simulink model "tt_sim"  (R2018b)
settings: Solver=FixedStepAuto  StartTime=0.0  StopTime=400  FixedStep=0.0001  RelTol=1e-5  EnableMultiTasking=on
StopFcn:
  | %e_unicycle_3d_trefoil_plot
libraries: simulink x2
settings Model: Creator=winston  LastModifiedBy=winston
settings SolverCC: AutoInsertRateTranBlk=on
settings DataIOCC: SaveOutput=off  SignalLogging=off  DSMLogging=off  SaveTime=off
settings OptimizationCC: LifeSpan=inf
settings DebuggingCC: AllowSymbolicDim=off  LibraryContextMissingDiagnostic=none  SFUnexpectedBacktrackingDiag=warning  SFNoUnconditionalDefaultTransitionDiag=warning  SFExecutionAtInitializationDiag=none  UnderSpecifiedDimensionMsg=warning
settings ModelReferenceCC: PropagateSignalLabelsOutOfModel=off
settings SFSimCC: SimUseLocalCustomCode=off
settings RTWCC: RTWUseLocalCustomCode=off
settings CodeAppCC: StateflowObjectComments=on
settings GRTTargetCC: TargetLangStandard=C89/C90 (ANSI)
settings ConfigComp: CovMetricSettings=dw  CovHtmlReporting=on  CovSaveCumulativeToWorkspaceVar=on  CovSaveSingleToWorkspaceVar=on  CovExternalEMLEnable=off

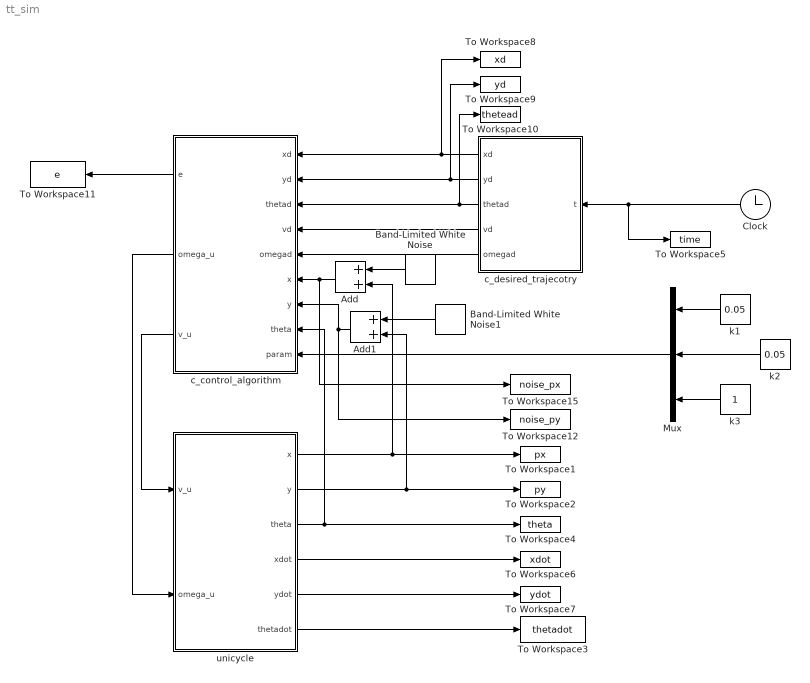
== system tt_sim ==
  Add : Sum
  Add1 : Sum
  Band-Limited White Noise : simulink/Sources/Band-Limited White Noise  Cov=10  Ts=0.1  seed=[23341]
  Band-Limited White Noise1 : simulink/Sources/Band-Limited White Noise  Cov=10  Ts=0.1  seed=[23]
  Clock : Clock
  Mux : Mux  Inputs=3
  To Workspace1 : ToWorkspace  VariableName=px  SampleTime=-1
  To Workspace10 : ToWorkspace  VariableName=thetead  SampleTime=-1
  To Workspace11 : ToWorkspace  VariableName=e  SaveFormat=Timeseries  SampleTime=-1
  To Workspace12 : ToWorkspace  VariableName=noise_py  SampleTime=-1
  To Workspace15 : ToWorkspace  VariableName=noise_px  SampleTime=-1
  To Workspace2 : ToWorkspace  VariableName=py  SampleTime=-1
  To Workspace3 : ToWorkspace  VariableName=thetadot  SampleTime=-1
  To Workspace4 : ToWorkspace  VariableName=theta  SampleTime=-1
  To Workspace5 : ToWorkspace  VariableName=time  SampleTime=-1
  To Workspace6 : ToWorkspace  VariableName=xdot  SampleTime=-1
  To Workspace7 : ToWorkspace  VariableName=ydot  SampleTime=-1
  To Workspace8 : ToWorkspace  VariableName=xd  SampleTime=-1
  To Workspace9 : ToWorkspace  VariableName=yd  SampleTime=-1
  c_control_algorithm : MATLAB Function  TreatAsAtomicUnit=on
  c_desired_trajecotry : MATLAB Function  TreatAsAtomicUnit=on
  k1 : Constant  Value=0.05
  k2 : Constant  Value=0.05
  k3 : Constant
  unicycle : Subsystem  mask{x0=300, y0=300, theta0=0}
      mask prompts: x0 "x(0)"; y0 "y(0)"; theta0 "theta(0)"
  wires:
  Mux/1 -> c_control_algorithm/9(param)
  c_control_algorithm/3(v_u) -> unicycle/1(v_u)
  c_control_algorithm/2(omega_u) -> unicycle/2(omega_u)
  k1/1 -> Mux/1
  k2/1 -> Mux/2
  k3/1 -> Mux/3
  Clock/1 -> To Workspace5/1, c_desired_trajecotry/1(t)
  unicycle/3(theta) -> c_control_algorithm/8(theta), To Workspace4/1
  unicycle/4(xdot) -> To Workspace6/1
  unicycle/5(ydot) -> To Workspace7/1
  unicycle/6(thetadot) -> To Workspace3/1
  c_desired_trajecotry/1(xd) -> c_control_algorithm/1(xd), To Workspace8/1
  c_desired_trajecotry/2(yd) -> c_control_algorithm/2(yd), To Workspace9/1
  c_desired_trajecotry/3(thetad) -> To Workspace10/1, c_control_algorithm/3(thetad)
  c_desired_trajecotry/4(vd) -> c_control_algorithm/4(vd)
  c_desired_trajecotry/5(omegad) -> c_control_algorithm/5(omegad)
  c_control_algorithm/1(e) -> To Workspace11/1
  unicycle/1(x) -> Add/2, To Workspace1/1
  Band-Limited White Noise/1 -> Add/1
  Add/1 -> To Workspace15/1, c_control_algorithm/6(x)
  unicycle/2(y) -> Add1/2, To Workspace2/1
  Band-Limited White Noise1/1 -> Add1/1
  Add1/1 -> c_control_algorithm/7(y), To Workspace12/1

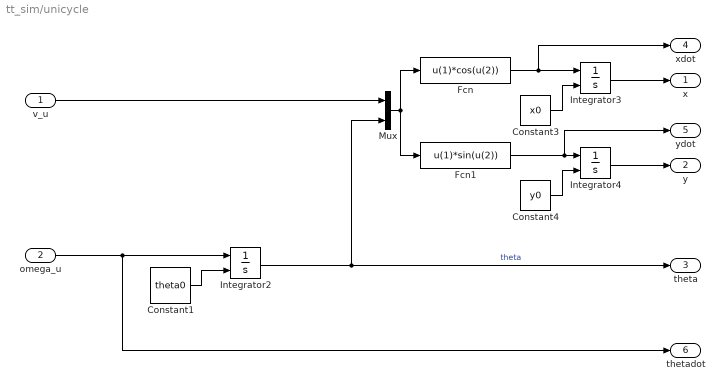
== system tt_sim/unicycle ==
  v_u : Inport
  omega_u : Inport  Port=2
  Constant1 : Constant  Value=theta0
  Constant3 : Constant  Value=x0
  Constant4 : Constant  Value=y0
  Fcn : Fcn  Expr=u(1)*cos(u(2))
  Fcn1 : Fcn  Expr=u(1)*sin(u(2))
  Integrator2 : Integrator  InitialConditionSource=external
  Integrator3 : Integrator  InitialConditionSource=external
  Integrator4 : Integrator  InitialConditionSource=external
  Mux : Mux  Inputs=2
  x : Outport
  y : Outport  Port=2
  theta : Outport  Port=3
  xdot : Outport  Port=4
  ydot : Outport  Port=5
  thetadot : Outport  Port=6
  wires:
  v_u/1 -> Mux/1
  Integrator2/1 -> theta/1, Mux/2  "theta"
  Mux/1 -> Fcn/1, Fcn1/1
  Fcn/1 -> xdot/1, Integrator3/1
  Fcn1/1 -> ydot/1, Integrator4/1
  Constant1/1 -> Integrator2/2
  Constant3/1 -> Integrator3/2
  Constant4/1 -> Integrator4/2
  omega_u/1 -> thetadot/1, Integrator2/1
  Integrator3/1 -> x/1
  Integrator4/1 -> y/1

== matlab function tt_sim/c_control_algorithm ==
  data: e output; omega_u output; xd input; yd input; thetad input; vd input; omegad input; v_u output; x input; y input; theta input; param input
function [e, omega_u, v_u] = fcn(xd, yd, thetad, vd, omegad, x, y, theta, param)
k1 = param(1); k2 = param(2); k3 = param(3);

M = [cos(theta), sin(theta), 0;
    -sin(theta), cos(theta), 0;
    0,           0         , 1];
e = M * [xd-x; yd-y; thetad-theta];

u1 = -k1*e(1);

tmp = sin(e(3))/e(3);
if(e(3) < 0.01)
    tmp = 1;
end
u2 = -k2*vd*e(2)*tmp - k3*e(3);

v_u = vd*cos(e(3)) - u1;
omega_u = omegad - u2;

== matlab function tt_sim/c_desired_trajecotry ==
  settings: updateMethod=DISCRETE
  data: t input; xd output; yd output; thetad output; vd output; omegad output
function [xd, yd, thetad, vd, omegad] = fcn(t)
persistent last_thetad
persistent unwrap_num
if isempty(last_thetad)
        last_thetad = 0;
end
if isempty(unwrap_num)
        unwrap_num = 0;
end

gain = 1/50; nx=3; ny=4; betax=0.1; betay=0.7;
xd = 250*cos(gain*nx*t+betax)+600;
yd = 250*cos(gain*ny*t+betay)+350;

dotxd = -15*sin((3*t)/50 + 1/10);
dotyd = -20*sin((2*t)/25 + 7/10);
thetad = atan2(dotyd, dotxd) + unwrap_num*2*pi;

% this part is to prevent discontinuity of atant2
if(thetad - last_thetad > pi)
    thetad = thetad-2*pi;
    unwrap_num = unwrap_num-1;
else
    if((thetad - last_thetad < -pi))
        thetad = thetad+2*pi;
        unwrap_num = unwrap_num+1;
    end
end
last_thetad = thetad;

vd = 5*(16*sin((2*t)/25 + 7/10)^2 + 9*sin((3*t)/50 + 1/10)^2)^(1/2);
omegad = (42*sin(t/50 + 3/5) - 6*sin((7*t)/50 + 4/5))/(225*cos((3*t)/25 + 1/5) + 400*cos((4*t)/25 + 7/5) - 625);
